simulink model "final_project"  (R2020b)
settings: Solver=VariableStepAuto  StartTime=0.0  StopTime=10.0  RelTol=1e-3
libraries: truetime x4
settings Model: Creator=ec  LastModifiedBy=ec

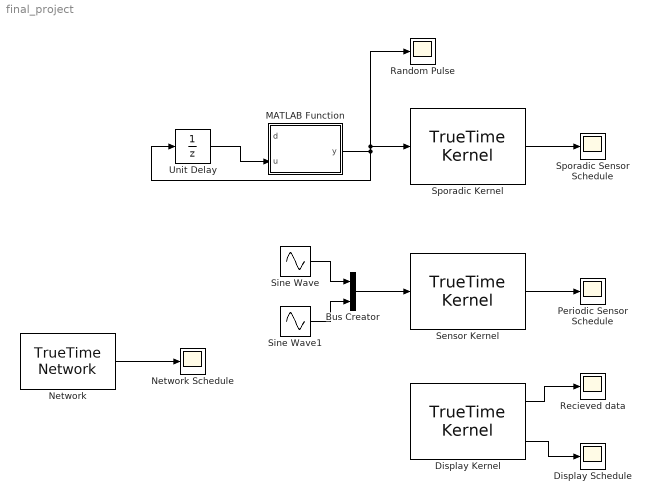
== system final_project ==
  Bus Creator : BusCreator  Inputs=2
  Display Kernel : truetime/TrueTime Kernel  sfun=display_kernel_init  args=[]  ninputsoutputs=[0 3]  ntriggers=0  trigtype=falling  nwnodenbr=[1 3]  clockoffsetdrift=[0 0]  schedoutput=on  battery=off  poweroutput=off  label=1: 3
  Display Schedule : Scope
  MATLAB Function : MATLAB Function  TreatAsAtomicUnit=on
  Network : truetime/TrueTime Network  nwtype=CSMA/CD (Ethernet)  nwnbr=1  nnodes=3  rate=1000000  minsize=32  lossprob=0  seed=0  bandwidths=[0.333 0.333 0.333]  slotsize=512  schedule=[1 1 2]  memsize=80000  buftype=Common buffer  overflow=Retransmit  dynSchedule=0  miniSlotSize=0  NIT=0  QSortMode=FIFO  sync=0  irtSchedule=0  nrtLength=0  nodeGraph=0  scheduleoutput=on
  Network Schedule : Scope
  Periodic Sensor Schedule : Scope
  Random Pulse : Scope
  Recieved data : Scope
  Sensor Kernel : truetime/TrueTime Kernel  sfun=periodic_kernel_init  args=[]  ninputsoutputs=[2 0]  ntriggers=0  trigtype=falling  nwnodenbr=[1 1]  clockoffsetdrift=[0 0]  schedoutput=on  battery=off  poweroutput=off  label=1: 1
  Sine Wave : Sin  Frequency=314.16  SampleTime=0
  Sine Wave1 : Sin  Frequency=754  SampleTime=0
  Sporadic Kernel : truetime/TrueTime Kernel  sfun=sporadic_kernel_init  args=[]  ninputsoutputs=[0 0]  ntriggers=1  trigtype=rising  nwnodenbr=[1 2]  clockoffsetdrift=[0 0]  schedoutput=on  battery=off  poweroutput=off  label=1: 2
  Sporadic Sensor Schedule : Scope
  Unit Delay : UnitDelay  SampleTime=-1  HasFrameUpgradeWarning=on
  wires:
  Network/1 -> Network Schedule/1
  Sensor Kernel/1 -> Periodic Sensor Schedule/1
  Display Kernel/2 -> Display Schedule/1
  Bus Creator/1 -> Sensor Kernel/1
  Sine Wave/1 -> Bus Creator/1
  Sine Wave1/1 -> Bus Creator/2
  Display Kernel/1 -> Recieved data/1
  Sporadic Kernel/1 -> Sporadic Sensor Schedule/1
  Unit Delay/1 -> MATLAB Function/2(u)
  MATLAB Function/1(y) -> Random Pulse/1, Sporadic Kernel/1, Unit Delay/1

== matlab function final_project/MATLAB Function ==
  data: d input; u input; y output
function y = fcn(d,u)
%#codegen
id=rand(1)
if id>d & u==0
  y=1
else
  y=0
end
